simulink model "DC_Motor"  (R2020b)
settings: Solver=VariableStepAuto  StartTime=0.0  StopTime=tTot  FixedStep=TsSim  RelTol=1e-6  EnableMultiTasking=on
InitFcn:
  | motor_init
StopFcn:
  | motor_plot
values from neighbouring files (symbols this model uses):
  Bm = 6.8e-4    (= 0.00068)    [motor_init.m]
  Jm = 0.00034    [LEGO_motor_init.m]    (also in motor_init.m = 0.002189)
  Kb = 0.5730    (= 0.573)    [motor_init.m]
  Km = 0.5791    [motor_init.m]
  L = 5.4e-3    (= 0.0054)    [motor_init.m]
  R = 1.45    [motor_init.m]
  TqDist = 0.055    [LEGO_motor_init.m]    (also in motor_init.m = 2.43)
  tStep = 0.0    (= 0)    [LEGO_motor_init.m]    (also in motor_init.m = 0.1)
  VStep = 90    [motor_init.m]
settings Model: Creator=Pixelated  LastModifiedBy=U00EBN1
settings DataIOCC: ReturnWorkspaceOutputs=off
settings OptimizationCC: LifeSpan=inf
settings DebuggingCC: IgnoredZcDiagnostic=none  SFUnexpectedBacktrackingDiag=warning  SFNoUnconditionalDefaultTransitionDiag=warning  SFExecutionAtInitializationDiag=none  ArithmeticOperatorsInVariantConditions=warning
settings SFSimCC: SimUseLocalCustomCode=off  CustomCodeUndefinedFunction=UseInterfaceOnly
settings RTWCC: RTWUseLocalCustomCode=off
settings CodeAppCC: StateflowObjectComments=on
settings GRTTargetCC: TargetLangStandard=C89/C90 (ANSI)
settings ConfigComp: CovMetricSettings=dw  CovSaveCumulativeToWorkspaceVar=on  CovSaveSingleToWorkspaceVar=on  CovExternalEMLEnable=off

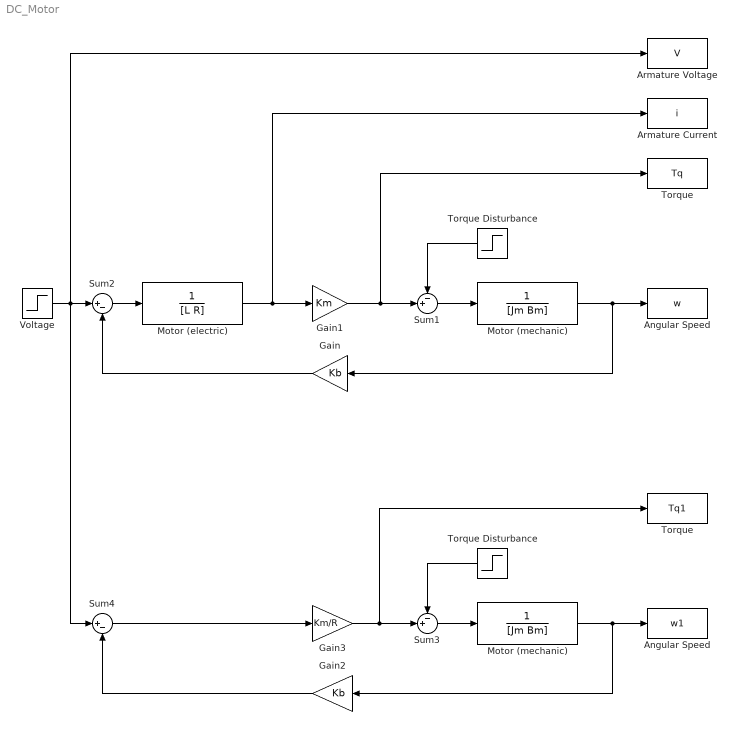
== system DC_Motor ==
  Angular Speed : ToWorkspace  VariableName=w  SampleTime=-1
  "Angular Speed " : ToWorkspace  VariableName=w1  SampleTime=-1
  Armature Current : ToWorkspace  VariableName=i  SampleTime=-1
  Armature Voltage : ToWorkspace  VariableName=V  SampleTime=-1
  Gain : Gain  Gain=Kb
  Gain1 : Gain  Gain=Km
  Gain2 : Gain  Gain=Kb
  Gain3 : Gain  Gain=Km/R
  Motor (electric) : TransferFcn  Denominator=[L R]
  Motor (mechanic) : TransferFcn  Denominator=[Jm Bm]
  "Motor (mechanic) " : TransferFcn  Denominator=[Jm Bm]
  Sum1 : Sum  Inputs=-+|
  Sum2 : Sum  Inputs=|+-
  Sum3 : Sum  Inputs=-+|
  Sum4 : Sum  Inputs=|+-
  Torque : ToWorkspace  VariableName=Tq  SampleTime=-1
  "Torque " : ToWorkspace  VariableName=Tq1  SampleTime=-1
  Torque Disturbance : Step  Time=tStep  After=TqDist  SampleTime=0
  "Torque Disturbance " : Step  Time=tStep  After=TqDist  SampleTime=0
  Voltage : Step  Time=tStep  After=VStep  SampleTime=0
  wires:
  Motor (mechanic)/1 -> Angular Speed/1, Gain/1
  Sum2/1 -> Motor (electric)/1
  Voltage/1 -> Sum4/1, Armature Voltage/1, Sum2/1
  Gain/1 -> Sum2/2
  Motor (electric)/1 -> Armature Current/1, Gain1/1
  Sum1/1 -> Motor (mechanic)/1
  Torque Disturbance/1 -> Sum1/1
  "Torque Disturbance "/1 -> Sum3/1
  Gain3/1 -> "Torque "/1, Sum3/2
  Sum4/1 -> Gain3/1
  Sum3/1 -> "Motor (mechanic) "/1
  Gain2/1 -> Sum4/2
  "Motor (mechanic) "/1 -> "Angular Speed "/1, Gain2/1
  Gain1/1 -> Torque/1, Sum1/2
